simulink model "Inner1"  (Simulink 5.0)
settings: Solver=ode45  StartTime=0.0  StopTime=10.0  RelTol=1e-3
undefined symbols (not defined in the file): sigbuilder_block
settings Model: Creator=scaife  LastModifiedBy=scaife  ExtModeAutoUpdateStatusClock=off

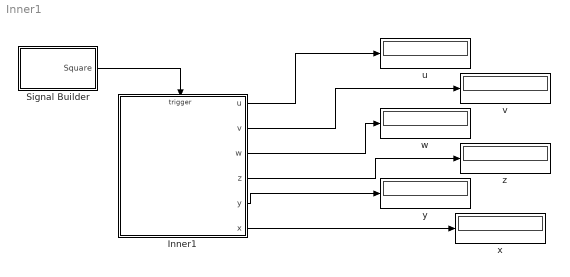
== system Inner1 ==
  Inner1 : Stateflow chart
  Signal Builder : Subsystem  Tag=STV Subsys  StartFcn=sigbuilder_block('start');  StopFcn=sigbuilder_block('stop');  ClipboardFcn=sigbuilder_block('clipboard');  mask(Sigbuilder block){}
      mask help: Sigbuilder GUI
      mask init:
      | if ~strcmp(get_param(bdroot(gcb),'SimulationStatus'),'stopped') tuvar = sigbuilder_block('maskInit'); end
      settings: CopyFcn=sigbuilder_block('copy');  DeleteFcn=sigbuilder_block('delete');  ModelCloseFcn=sigbuilder_block('modelClose');  PreSaveFcn=sigbuilder_block('preSave');  NameChangeFcn=sigbuilder_block('namechange');  OpenFcn=sigbuilder_block('open',[50 50 520 400 ]);  CloseFcn=sigbuilder_block('close');
      mask Display: plot(0,0,100,100,[10,10,40,40,10],[80,20,20,80,80],[40,10],[50,50], [40,27,10],[65,72,56],[40,25,25,10],[28,28,43,43]);
  u : Display
  v : Display
  w : Display
  x : Display
  y : Display
  z : Display
  wires:
  Signal Builder/1(Square) -> Inner1/Trigger
  Inner1/1(u) -> u/1
  Inner1/2(v) -> v/1
  Inner1/3(w) -> w/1
  Inner1/4(z) -> z/1
  Inner1/5(y) -> y/1
  Inner1/6(x) -> x/1

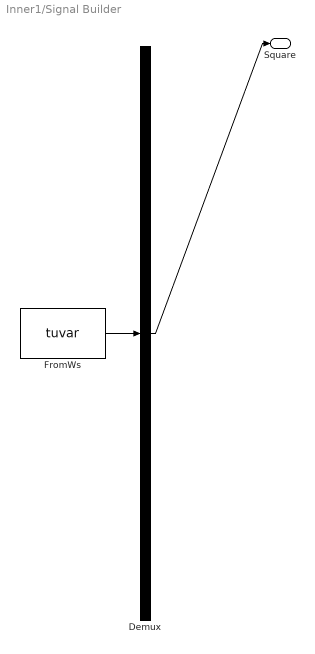
== system Inner1/Signal Builder ==
  Demux : Demux  Tag=STV Demux  Outputs=1
  FromWs : FromWorkspace  Tag=STV FromWs  VariableName=tuvar  SampleTime=0  SigBuilderData=DataTag0
  Square : Outport  Tag=STV Outport
  wires:
  FromWs/1 -> Demux/1
  Demux/1 -> Square/1

== stateflow chart Inner1 ==
  state A/
    du: u++;
    state A1/
      en: x+=1;
      du: x+=10;
    state A2/
      en: x+=1000;
      du: x+=10000;
    state A3/
      ex: v+=1000;
      state A3a/
        ex: v+=10000;
      (default) -> A3a
    A -> A1 : E[u%%3==0]{y++;}/z++;
    A -> (junction 8) : E[u%%3==2]{w++;}/v++;
    A -> A2 : E[u%%3==1]
        | {y+=1000;}/z+=1000;
    (default) -> A3
  (default) -> A
  data: u output int32; v output int32; w output int32; z output int32; y output int32; x output int32
  events: E input EITHER_EDGE_EVENT
